simulink model "aftc_architecture_model"  (R2024a)
settings: Solver=VariableStepAuto  StartTime=0.0  StopTime=10.0  RelTol=1e-3
settings Model: Creator=Admin  LastModifiedBy=Admin

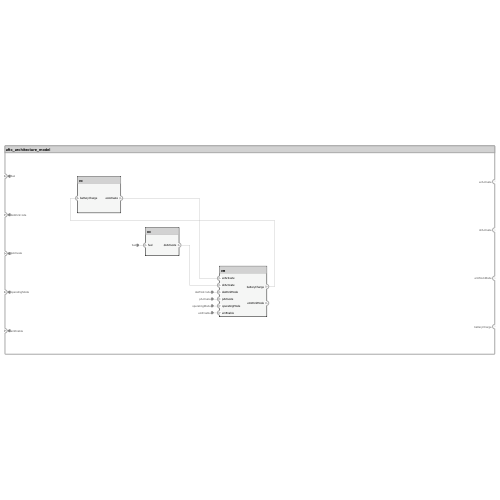
[thumbnail: Simulink's stored preview of the top-level diagram]
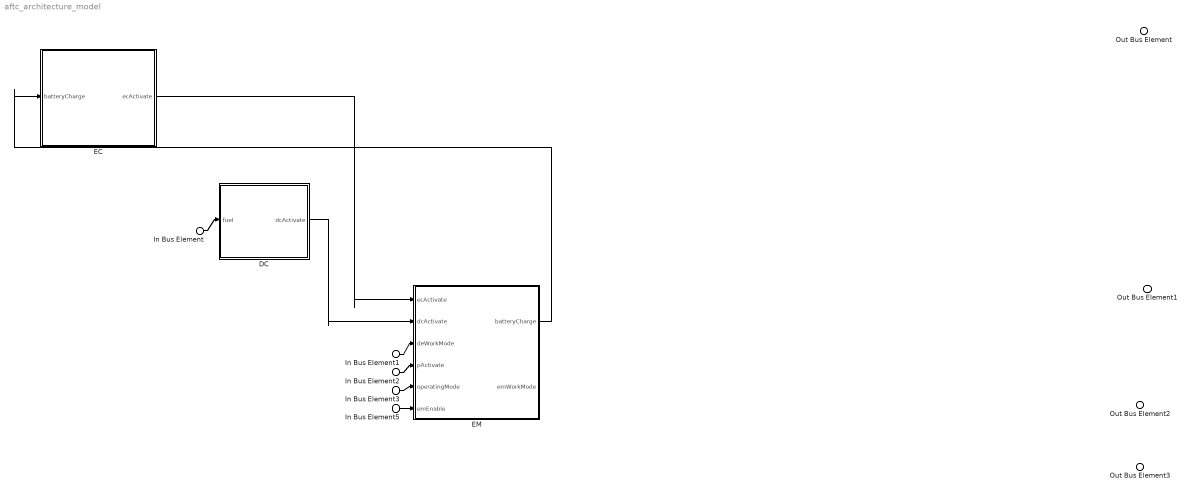
== system aftc_architecture_model ==
  In Bus Element : Inport  PortName=fuel
  In Bus Element1 : Inport  Port=2  PortName=deWork<ode
  In Bus Element2 : Inport  Port=3  PortName=pActivate
  In Bus Element3 : Inport  Port=4  PortName=operatingMode
  In Bus Element5 : Inport  Port=5  PortName=emEnable
  DC : Subsystem
      settings: PortSchema="{\"entries\":[{\"content\":{\"headerSize\":26,\"margin\":15,\"minimumSpacing\":25,\"sides\":[{\"content\":{\"connectorIds\":[\"In1\"]},\"type\":\"ConnectorPlacement.EquallySpacedRectSide\",\"uuid\":\"6cd64777-7118-4da3-a4e3-1f769f1ba9ff\"},{\"content\":{\"connectorIds\":[\"Out1\"],\"side\":\"RIGHT\"},\"type\":\"ConnectorPlacement.EquallySpacedRectSide\",\"uuid\":\"07320f2b-f593-407a-9be8-f5c69e458813\"},{\"content\":{\"side\":\"TOP\"},\"type\":\"ConnectorPlacement.EquallySpacedRectSide\",\"uuid\":\"3b066712-d361-493e-aaf9-f8d607354b36\"}]},\"type\":\"ConnectorPlacement.EquallySpacedConnector\",\"uuid\":\"26a06246-8dfb-4dbb-a982-17c9b4b0327d\"}],\"packageUris\":[\"http://schema.mathworks.com/mf0/Connector/R2020b\"],\"version\":\"1.0\"}"
  EC : Subsystem
      settings: PortSchema="{\"entries\":[{\"content\":{\"headerSize\":26,\"margin\":15,\"minimumSpacing\":25,\"sides\":[{\"content\":{\"connectorIds\":[\"In1\"]},\"type\":\"ConnectorPlacement.EquallySpacedRectSide\",\"uuid\":\"6cd64777-7118-4da3-a4e3-1f769f1ba9ff\"},{\"content\":{\"connectorIds\":[\"Out1\"],\"side\":\"RIGHT\"},\"type\":\"ConnectorPlacement.EquallySpacedRectSide\",\"uuid\":\"07320f2b-f593-407a-9be8-f5c69e458813\"},{\"content\":{\"side\":\"TOP\"},\"type\":\"ConnectorPlacement.EquallySpacedRectSide\",\"uuid\":\"3b066712-d361-493e-aaf9-f8d607354b36\"}]},\"type\":\"ConnectorPlacement.EquallySpacedConnector\",\"uuid\":\"26a06246-8dfb-4dbb-a982-17c9b4b0327d\"}],\"packageUris\":[\"http://schema.mathworks.com/mf0/Connector/R2020b\"],\"version\":\"1.0\"}"
  EM : Subsystem
      settings: PortSchema="{\"entries\":[{\"content\":{\"headerSize\":26,\"margin\":15,\"minimumSpacing\":25,\"sides\":[{\"content\":{\"connectorIds\":[\"In1\",\"In2\",\"In3\",\"In4\",\"In5\",\"In6\"]},\"type\":\"ConnectorPlacement.EquallySpacedRectSide\",\"uuid\":\"6cd64777-7118-4da3-a4e3-1f769f1ba9ff\"},{\"content\":{\"connectorIds\":[\"Out1\",\"Out2\"],\"side\":\"RIGHT\"},\"type\":\"ConnectorPlacement.EquallySpacedRectSide\",\"uuid\":\"07320f2b-f593-407a-9be8-f5c69e458813\"},{\"content\":{\"side\":\"TOP\"},\"type\":\"ConnectorPlacement.EquallySpacedRectSide\",\"uuid\":\"3b066712-d361-493e-aaf9-f8d607354b36\"}]},\"type\":\"ConnectorPlacement.EquallySpacedConnector\",\"uuid\":\"26a06246-8dfb-4dbb-a982-17c9b4b0327d\"}],\"packageUris\":[\"http://schema.mathworks.com/mf0/Connector/R2020b\"],\"version\":\"1.0\"}"
  Out Bus Element : Outport  PortName=ecActivate
  Out Bus Element1 : Outport  Port=2  PortName=dcActivate
  Out Bus Element2 : Outport  Port=3  PortName=emWorkMode
  Out Bus Element3 : Outport  Port=4  PortName=batteryCharge
  wires:
  In Bus Element/1 -> DC/1(fuel)
  EM/1(batteryCharge) -> EC/1(batteryCharge)
  In Bus Element1/1 -> EM/3(deWorkMode)
  In Bus Element2/1 -> EM/4(pActivate)
  In Bus Element3/1 -> EM/5(operatingMode)
  In Bus Element5/1 -> EM/6(emEnable)
  EC/1(ecActivate) -> EM/1(ecActivate)
  DC/1(dcActivate) -> EM/2(dcActivate)

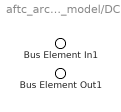
== system aftc_architecture_model/DC ==
  Bus Element In1 : Inport  PortName=fuel
  Bus Element Out1 : Outport  PortName=dcActivate

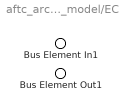
== system aftc_architecture_model/EC ==
  Bus Element In1 : Inport  PortName=batteryCharge
  Bus Element Out1 : Outport  PortName=ecActivate

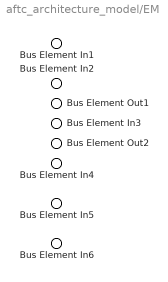
== system aftc_architecture_model/EM ==
  Bus Element In1 : Inport  PortName=ecActivate
  Bus Element In2 : Inport  Port=2  PortName=dcActivate
  Bus Element In3 : Inport  Port=3  PortName=deWorkMode
  Bus Element In4 : Inport  Port=4  PortName=pActivate
  Bus Element In5 : Inport  Port=5  PortName=operatingMode
  Bus Element In6 : Inport  Port=6  PortName=emEnable
  Bus Element Out1 : Outport  PortName=batteryCharge
  Bus Element Out2 : Outport  Port=2  PortName=emWorkMode
